simulink model "Example_5_3"  (R2021b)
settings: Solver=VariableStepAuto  StartTime=0.0  StopTime=10.0  RelTol=1e-3
settings Model: Creator=Living Dead!  LastModifiedBy=saeed
settings DebuggingCC: UnconnectedInputMsg=none  UnconnectedOutputMsg=none  UnconnectedLineMsg=none
settings ModelReferenceCC: EnableRefExpFcnMdlSchedulingChecks=off
settings RTWCC: GPUComputeCapability=5.0  DLArmComputeVersion=20.02.1

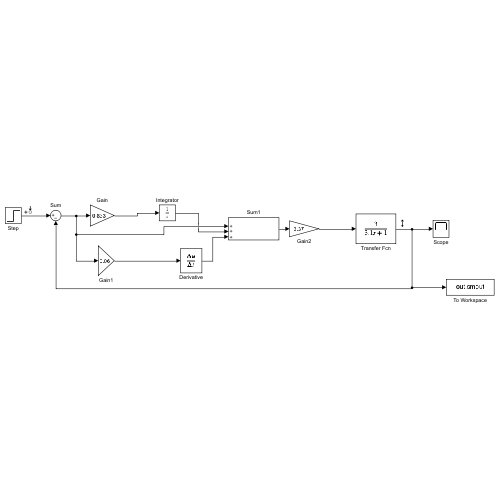
[thumbnail: Simulink's stored preview of the top-level diagram]
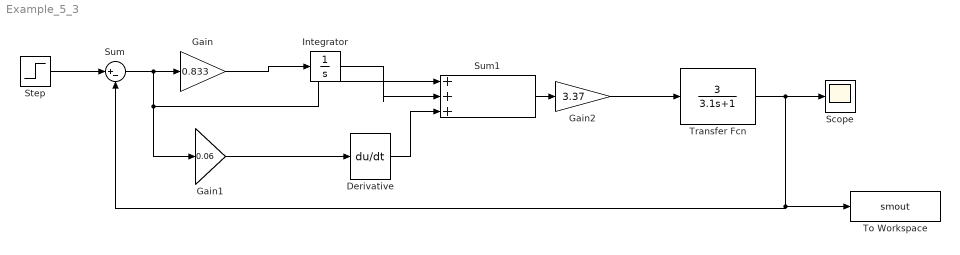
== system Example_5_3 ==
  Derivative : Derivative
  Gain : Gain  Gain=0.833
  Gain1 : Gain  Gain=0.06
  Gain2 : Gain  Gain=3.37
  Integrator : Integrator
  Scope : Scope
  Step : Step  Time=0  After=30  SampleTime=0
  Sum : Sum  Inputs=|+-
  Sum1 : Sum  Inputs=|+++
  To Workspace : ToWorkspace  VariableName=smout  SaveFormat=Timeseries  SampleTime=-1
  Transfer Fcn : TransferFcn  Numerator=[3]  Denominator=[3.1 1]
  wires:
  Step/1 -> Sum/1
  Gain/1 -> Integrator/1
  Gain2/1 -> Transfer Fcn/1
  Derivative/1 -> Sum1/3
  Integrator/1 -> Sum1/2
  Sum/1 -> Gain1/1, Sum1/1, Gain/1
  Sum1/1 -> Gain2/1
  Gain1/1 -> Derivative/1
  Transfer Fcn/1 -> Scope/1, To Workspace/1, Sum/2
